simulink model "testReactionWheel"  (R2021a)
settings: Solver=VariableStepAuto  StartTime=0.0  StopTime=Torb  RelTol=1e-3
values from neighbouring files (symbols this model uses):
  t0 = 1000    [dynamics_2.m]
  tramp = 10    [dynamics_2.m]
  twait = 10*pi/wz0    [dynamics_2.m]
  wzrw = (Isc(3,3) + Irw(3,3))/Irw(3,3)* wz0    [dynamics_2.m]
libraries: simulink x4, sharedtransform x1
settings Model: DataDictionary=databus.sldd  Creator=Laura  LastModifiedBy=Laura

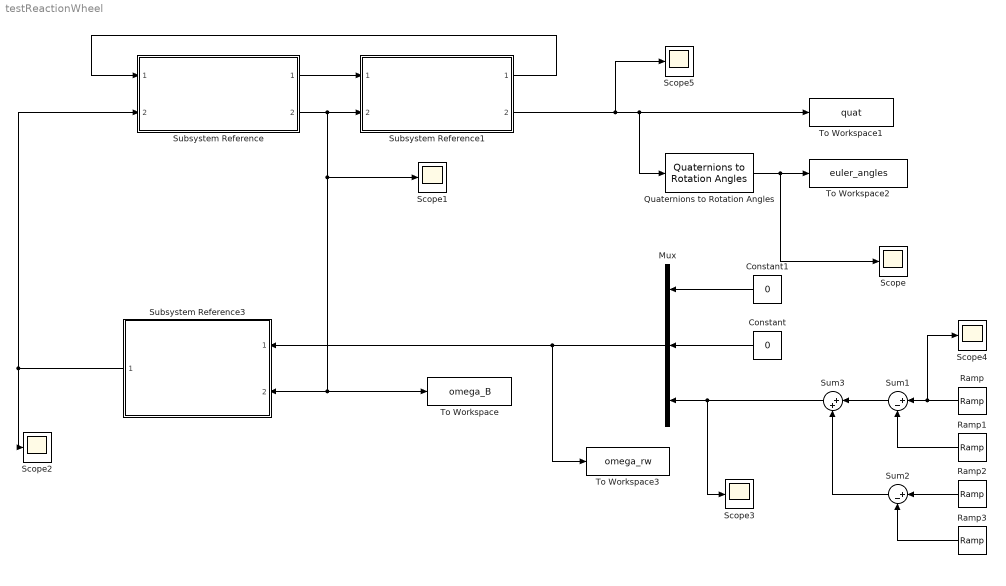
== system testReactionWheel ==
  Constant : Constant  Value=0
  Constant1 : Constant  Value=0
  Mux : Mux  Inputs=3
  Quaternions to Rotation Angles : sharedtransform/Quaternions to Rotation Angles  rotationOrder=ZYX  aMode=aMode
      settings: SourceProductBaseCode=AE,PW,DR,MT,UV,VE
  Ramp : simulink/Sources/Ramp  slope=wzrw/tramp  start=t0  InitialOutput=0
  Ramp1 : simulink/Sources/Ramp  slope=wzrw/tramp  start=t0+tramp  InitialOutput=0
  Ramp2 : simulink/Sources/Ramp  slope=-wzrw/tramp  start=t0+twait  InitialOutput=0
  Ramp3 : simulink/Sources/Ramp  slope=-wzrw/(4010-4000)  start=t0+twait+tramp  InitialOutput=0
  Scope{,1..5} (6 alike) : Scope
  Subsystem Reference : Subsystem  ReferencedSubsystem=Dynamics
  Subsystem Reference1 : Subsystem  ReferencedSubsystem=Kinematics
  Subsystem Reference3 : Subsystem  ReferencedSubsystem=RWDynamics
  Sum1 : Sum  Inputs=|+-
  Sum2 : Sum  Inputs=|+-
  Sum3 : Sum  Inputs=|++
  To Workspace : ToWorkspace  VariableName=omega_B  SaveFormat=Timeseries  SampleTime=-1
  To Workspace1 : ToWorkspace  VariableName=quat  SaveFormat=Timeseries  SampleTime=-1
  To Workspace2 : ToWorkspace  VariableName=euler_angles  SaveFormat=Timeseries  SampleTime=-1
  To Workspace3 : ToWorkspace  VariableName=omega_rw  SaveFormat=Timeseries  SampleTime=-1
  wires:
  Quaternions to Rotation Angles/1 -> Scope/1, To Workspace2/1
  Subsystem Reference1/1 -> Subsystem Reference/1
  Subsystem Reference1/2 -> Scope5/1, To Workspace1/1, Quaternions to Rotation Angles/1
  Subsystem Reference/2 -> Scope1/1, Subsystem Reference3/2, To Workspace/1, Subsystem Reference1/2
  Subsystem Reference/1 -> Subsystem Reference1/1
  Subsystem Reference3/1 -> Scope2/1, Subsystem Reference/2
  Mux/1 -> To Workspace3/1, Subsystem Reference3/1
  Constant/1 -> Mux/2
  Constant1/1 -> Mux/1
  Ramp/1 -> Scope4/1, Sum1/1
  Ramp1/1 -> Sum1/2
  Ramp3/1 -> Sum2/2
  Ramp2/1 -> Sum2/1
  Sum3/1 -> Scope3/1, Mux/3
  Sum1/1 -> Sum3/1
  Sum2/1 -> Sum3/2
